simulink subsystem "ACS_Software"  (R2024a)
settings: Solver=VariableStepAuto  StartTime=0.0  StopTime=10.0  RelTol=1e-3
undefined symbols (not defined in the file): epoch, IAU, juliandate, k_Bdot, Kd, km, Kp, m, NoiseStd, s, signQuat, simulator, WMM2020
libraries: sharedtransform x15, simulink_extras x8, aerolibconvert2 x6, matrix_library x5, aerolibutil x5, aerolibtransform2 x2, sharedutil x1, SepehrMILLib x1, aerolibgravity2 x1
(part 1 of 2)
settings Model: Creator=dani  LastModifiedBy=dani

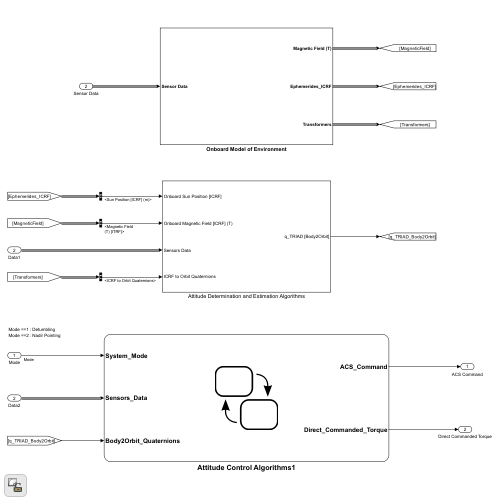
[thumbnail: Simulink's stored preview of the top-level diagram]
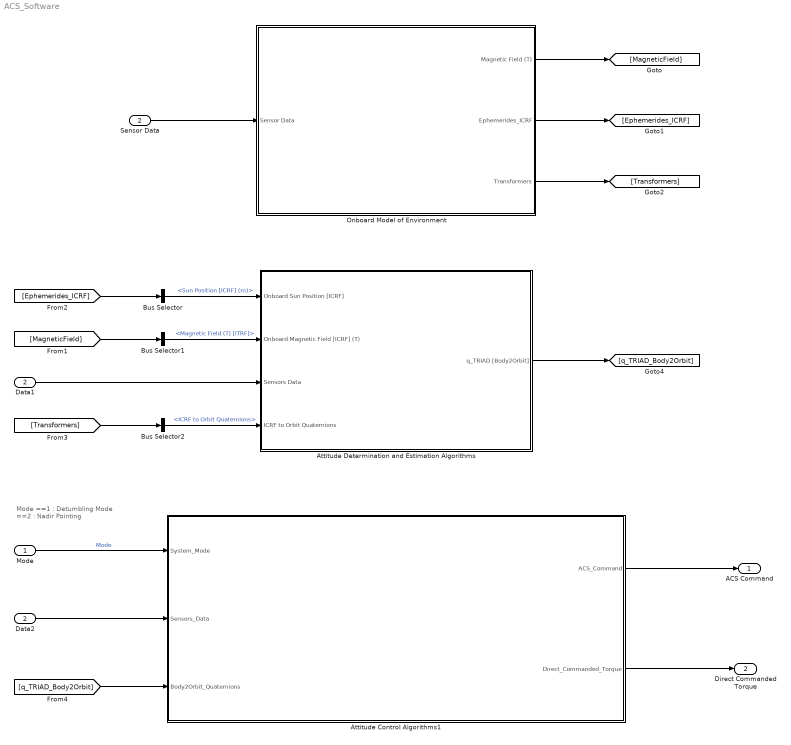
== system ACS_Software ==
  note: Mode ==1 : Detumbling
      | Mode ==2 : Nadir Pointing
  Mode : Inport
  Sensor Data : Inport  Port=2
  Attitude Control Algorithms1 : Stateflow chart  TreatAsAtomicUnit=on
  Attitude Determination and Estimation Algorithms : Subsystem
  Bus Selector : BusSelector  OutputSignals=Sun Ephemeris [ICRF].Sun Position [ICRF] (m)
  Bus Selector1 : BusSelector  OutputSignals=|
      | Magnetic Field
      | (T) [ITRF]
  Bus Selector2 : BusSelector  OutputSignals=Quaternions.ICRF to Orbit Quaternions
  Data1 : InportShadow  Port=2
  Data2 : InportShadow  Port=2
  Onboard Model of Environment : Subsystem
  ACS Command : Outport
  Direct Commanded Torque : Outport  Port=2
  wires:
  Attitude Determination and Estimation Algorithms/1(q_TRIAD [Body2Orbit]) -> [q_TRIAD_Body2Orbit]
  [MagneticField] -> Bus Selector1/1
  Onboard Model of Environment/1(Magnetic Field (T)) -> [MagneticField]
  [Ephemerides_ICRF] -> Bus Selector/1
  Onboard Model of Environment/2(Ephemerides_ICRF) -> [Ephemerides_ICRF]
  Sensor Data/1 -> Onboard Model of Environment/1(Sensor Data)
  Data1/1 -> Attitude Determination and Estimation Algorithms/3(Sensors Data)
  Mode/1 -> Attitude Control Algorithms1/1(System_Mode)  "Mode"
  Attitude Control Algorithms1/1(ACS_Command) -> ACS Command/1
  Data2/1 -> Attitude Control Algorithms1/2(Sensors_Data)
  Bus Selector/1 -> Attitude Determination and Estimation Algorithms/1(Onboard Sun Position [ICRF])  "<Sun Position [ICRF] (m)>"
  Bus Selector1/1 -> Attitude Determination and Estimation Algorithms/2(Onboard Magnetic Field [ICRF] (T))  "<Magnetic Field (T) [ITRF]>"
  Onboard Model of Environment/3(Transformers) -> [Transformers]
  [Transformers] -> Bus Selector2/1
  Bus Selector2/1 -> Attitude Determination and Estimation Algorithms/4(ICRF to Orbit Quaternions)  "<ICRF to Orbit Quaternions>"
  [q_TRIAD_Body2Orbit] -> Attitude Control Algorithms1/3(Body2Orbit_Quaternions)
  Attitude Control Algorithms1/2(Direct_Commanded_Torque) -> Direct Commanded Torque/1

== system ACS_Software/Attitude Control Algorithms1/Detumbling ==
  note: $\frac{k}{||B||}\omega \times B$
  Sensors_Data : Inport
  Action Port : ActionPort
      settings: CopyFcn=Stateflow.SLINSF.SimulinkMan.removeBlockPreDeleteFcn  PreDeleteFcn=Stateflow.SLINSF.SimulinkMan.unsafePredeleteFcn
  Bus Selector1 : BusSelector  OutputSignals=Measured Angular Velocity [Body] (rad/s),Measured Magnetic Field [Body] (T)
  Constant11 : Constant  Value=k_Bdot
  Cross Product : matrix_library/Cross Product
  Divide : Product  Inputs=*/
  Divide1 : Product  Inputs=*/
  Product : Product
  sqrt : Subsystem
  ACS_Command : Outport
  wires:
  sqrt/1(sqrt(u)) -> Divide1/2, Divide/2  "||B||"
  Constant11/1 -> Product/1
  Bus Selector1/2 -> sqrt/1(u), Divide/1  "<Measured Magnetic Field [Body] (T)>"
  Divide/1 -> Cross Product/2  "b"
  Bus Selector1/1 -> Cross Product/1  "<Measured Angular Velocity [Body] (rad/s)>"
  Sensors_Data/1 -> Bus Selector1/1
  Divide1/1 -> ACS_Command/1  "Dipole Command"
  Product/1 -> Divide1/1  "k(omega*b)"
  Cross Product/1 -> Product/2  "omega*b"

== system ACS_Software/Attitude Control Algorithms1/Nadir_Pointing ==
  System_Mode : Inport
  Sensors_Data : Inport  Port=2
  Body2Orbit_Quaternions : Inport  Port=3
  Action Port : ActionPort
      settings: CopyFcn=Stateflow.SLINSF.SimulinkMan.removeBlockPreDeleteFcn  PreDeleteFcn=Stateflow.SLINSF.SimulinkMan.unsafePredeleteFcn
  Nadir Pointing Algorithm : Subsystem
  Terminator : Terminator
  ACS_Command : Outport
  Direct_Commanded_Torque : Outport  Port=2
  wires:
  Sensors_Data/1 -> Nadir Pointing Algorithm/1(Sensors Out)
  Nadir Pointing Algorithm/1(Dipole Command) -> ACS_Command/1  "Dipole Command"
  System_Mode/1 -> Terminator/1
  Nadir Pointing Algorithm/2(Torque Command) -> Direct_Commanded_Torque/1  "Torque Command"
  Body2Orbit_Quaternions/1 -> Nadir Pointing Algorithm/2(Body to Orbit Quaternion)

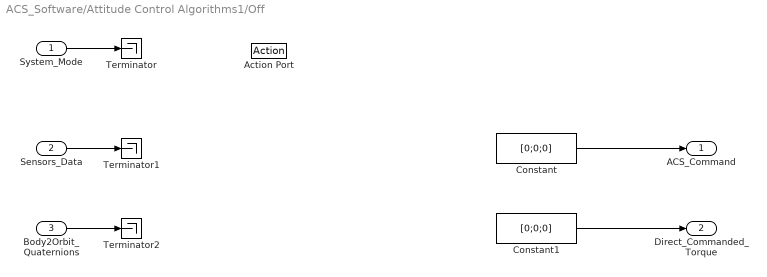
== system ACS_Software/Attitude Control Algorithms1/Off ==
  System_Mode : Inport
  Sensors_Data : Inport  Port=2
  Body2Orbit_Quaternions : Inport  Port=3
  Action Port : ActionPort
      settings: CopyFcn=Stateflow.SLINSF.SimulinkMan.removeBlockPreDeleteFcn  PreDeleteFcn=Stateflow.SLINSF.SimulinkMan.unsafePredeleteFcn
  Constant : Constant  Value=[0;0;0]
  Constant1 : Constant  Value=[0;0;0]
  Terminator : Terminator
  Terminator1 : Terminator
  Terminator2 : Terminator
  ACS_Command : Outport
  Direct_Commanded_Torque : Outport  Port=2
  wires:
  Sensors_Data/1 -> Terminator1/1
  System_Mode/1 -> Terminator/1
  Body2Orbit_Quaternions/1 -> Terminator2/1
  Constant/1 -> ACS_Command/1
  Constant1/1 -> Direct_Commanded_Torque/1

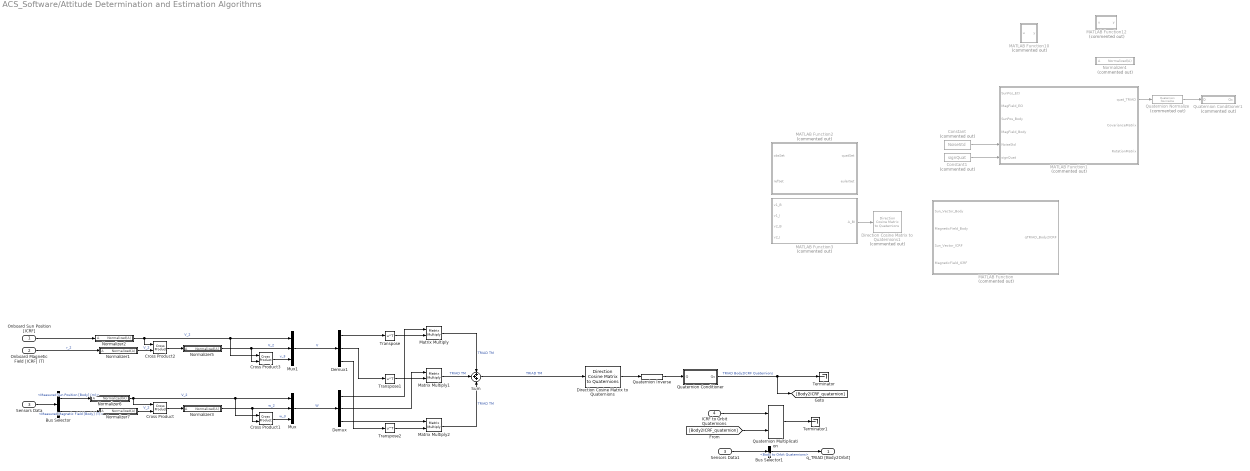
== system ACS_Software/Attitude Determination and Estimation Algorithms ==
  Onboard Sun Position [ICRF] : Inport
  Onboard Magnetic Field [ICRF] (T) : Inport  Port=2
  Sensors Data : Inport  Port=3
  ICRF to Orbit Quaternions : Inport  Port=4
  Bus Selector : BusSelector  OutputSignals=Measured Sun Position [Body] (m),Measured Magnetic Field [Body] (T)
  Bus Selector1 : BusSelector  OutputSignals=Body to Orbit Quaternions
  Constant : Constant  Commented=on  Value=NoiseStd
  Constant1 : Constant  Commented=on  Value=signQuat
  Cross Product{,1..3} (4 alike) : matrix_library/Cross Product
  Demux : Demux  Outputs=3
  Demux1 : Demux  Outputs=3
  Direction Cosine Matrix to Quaternions : sharedtransform/Direction Cosine Matrix  to Quaternions  aMode=0  action=None  tolerance=eps(2)
      settings: LibrarySourceBlock=|
      | aerolibtransform2/Direction Cosine Matrix
      | to Quaternions
  Direction Cosine Matrix to Quaternions1 : sharedtransform/Direction Cosine Matrix  to Quaternions  Commented=on  aMode=0  action=None  tolerance=eps(2)
      settings: LibrarySourceBlock=|
      | aerolibtransform2/Direction Cosine Matrix
      | to Quaternions
  MATLAB Function : MATLAB Function  Commented=on  TreatAsAtomicUnit=on
  MATLAB Function1 : MATLAB Function  Commented=on  TreatAsAtomicUnit=on
  MATLAB Function10 : MATLAB Function  Commented=on  TreatAsAtomicUnit=on
  MATLAB Function12 : MATLAB Function  Commented=on  TreatAsAtomicUnit=on
  MATLAB Function2 : MATLAB Function  Commented=on  TreatAsAtomicUnit=on
  MATLAB Function3 : MATLAB Function  Commented=on  TreatAsAtomicUnit=on
  Matrix Multiply : Product  Multiplication=Matrix(*)
  Matrix Multiply1 : Product  Multiplication=Matrix(*)
  Matrix Multiply2 : Product  Multiplication=Matrix(*)
  Mux : Mux  Inputs=3
  Mux1 : Mux  Inputs=3
  Normalizer1 : Subsystem
  Normalizer2 : Subsystem
  Normalizer3 : Subsystem
  Normalizer4 : Subsystem  Commented=on
  Normalizer5 : Subsystem
  Normalizer6 : Subsystem
  Normalizer7 : Subsystem
  Quaternion Inverse : aerolibutil/Quaternion Inverse
  Quaternion Multiplication : aerolibutil/Quaternion Multiplication
  Quaternion Normalize : sharedutil/Quaternion Normalize  Commented=on  aMode=aMode
  Quaternion Conditioner : Subsystem  TreatAsAtomicUnit=on
      settings: MinAlgLoopOccurrences=on
  Quaternion Conditioner1 : Subsystem  Commented=on  TreatAsAtomicUnit=on
      settings: MinAlgLoopOccurrences=on
  Sensors Data1 : InportShadow  Port=3
  Sum : Sum  Inputs=+++
  Terminator : Terminator
  Terminator1 : Terminator
  Transpose : Math  Operator=transpose
  Transpose1 : Math  Operator=transpose
  Transpose2 : Math  Operator=transpose
  q_TRIAD [Body2Orbit] : Outport
  wires:
  Bus Selector1/1 -> q_TRIAD [Body2Orbit]/1  "<Body to Orbit Quaternions>"
  Sensors Data1/1 -> Bus Selector1/1
  Quaternion Inverse/1 -> Quaternion Conditioner/1(Q)
  Quaternion Multiplication/1 -> Terminator1/1
  [Body2ICRF_quaternion] -> Quaternion Multiplication/2
  ICRF to Orbit Quaternions/1 -> Quaternion Multiplication/1
  Normalizer7/1(Normalized(A)) -> Cross Product/2  "V_2"
  Normalizer6/1(Normalized(A)) -> Mux/1, Cross Product1/1, Cross Product/1  "V_2"
  Normalizer2/1(Normalized(A)) -> Mux1/1, Cross Product3/1, Cross Product2/1  "V_2"
  Normalizer1/1(Normalized(A)) -> Cross Product2/2  "V_2"
  Bus Selector/1 -> Normalizer6/1(A)  "<Measured Sun Position [Body] (m)>"
  Onboard Sun Position [ICRF]/1 -> Normalizer2/1(A)
  Normalizer3/1(Normalized(A)) -> Cross Product1/2, Mux/2  "w_2"
  Onboard Magnetic Field [ICRF] (T)/1 -> Normalizer1/1(A)  "r_2"
  Direction Cosine Matrix to Quaternions/1 -> Quaternion Inverse/1
  Quaternion Conditioner/1(Qc) -> [Body2ICRF_quaternion], Terminator/1  "TRIAD Body2ICRF Quaternions"
  MATLAB Function3/1(A_BI) -> Direction Cosine Matrix to Quaternions1/1
  Matrix Multiply/1 -> Sum/1  "TRIAD TM"
  Matrix Multiply2/1 -> Sum/3  "TRIAD TM"
  Matrix Multiply1/1 -> Sum/2  "TRIAD TM"
  Demux1/1 -> Transpose/1
  Demux1/2 -> Transpose1/1
  Demux/2 -> Matrix Multiply1/1
  Demux1/3 -> Transpose2/1
  Demux/3 -> Matrix Multiply2/1
  Transpose2/1 -> Matrix Multiply2/2
  Transpose1/1 -> Matrix Multiply1/2
  Demux/1 -> Matrix Multiply/1
  Sum/1 -> Direction Cosine Matrix to Quaternions/1  "TRIAD TM"
  Transpose/1 -> Matrix Multiply/2
  Normalizer5/1(Normalized(A)) -> Mux1/2, Cross Product3/2  "V_2"
  Mux1/1 -> Demux1/1  "V"
  Cross Product3/1 -> Mux1/3  "v_3"
  Cross Product2/1 -> Normalizer5/1(A)
  Mux/1 -> Demux/1  "W"
  Cross Product1/1 -> Mux/3  "w_3"
  Cross Product/1 -> Normalizer3/1(A)
  Quaternion Normalize/1 -> Quaternion Conditioner1/1(Q)
  Constant1/1 -> MATLAB Function1/6(signQuat)
  Constant/1 -> MATLAB Function1/5(NoiseStd)
  Bus Selector/2 -> Normalizer7/1(A)  "<Measured Magnetic Field [Body] (T)>"
  Sensors Data/1 -> Bus Selector/1
  MATLAB Function1/1(quat_TRIAD) -> Quaternion Normalize/1

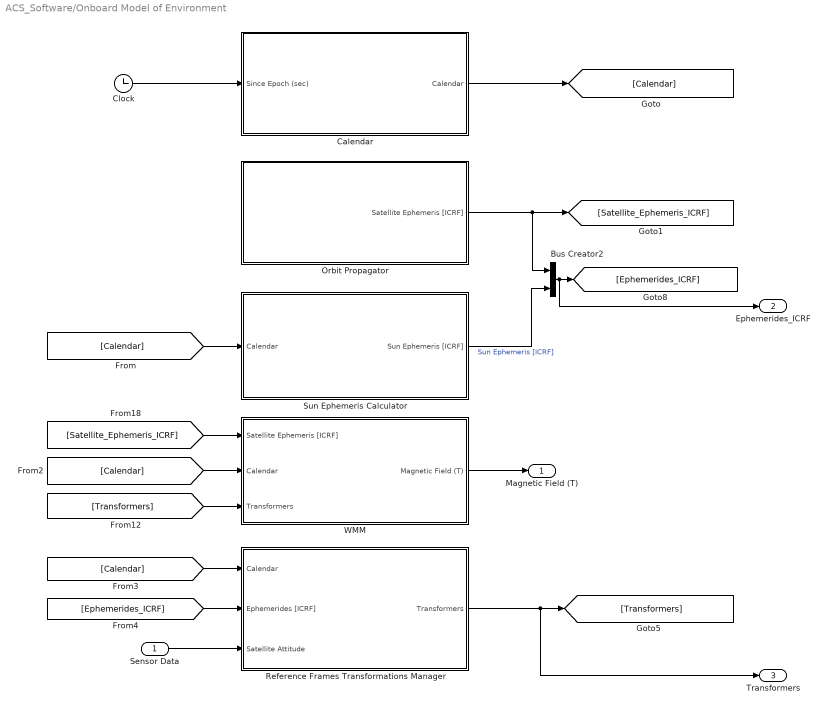
== system ACS_Software/Onboard Model of Environment ==
  Sensor Data : Inport
  Bus Creator2 : BusCreator  Inputs=2
  "Calendar " : Subsystem
  Clock : Clock
  Orbit Propagator : Subsystem
  Reference Frames Transformations Manager : Subsystem
  Sun Ephemeris Calculator : Subsystem
  WMM : Subsystem
  Magnetic Field (T) : Outport
  Ephemerides_ICRF : Outport  Port=2
  Transformers : Outport  Port=3
  wires:
  Sensor Data/1 -> Reference Frames Transformations Manager/3(Satellite Attitude)
  WMM/1(Magnetic Field (T)) -> Magnetic Field (T)/1
  Bus Creator2/1 -> [Ephemerides_ICRF], Ephemerides_ICRF/1
  [Ephemerides_ICRF] -> Reference Frames Transformations Manager/2(Ephemerides [ICRF])
  Clock/1 -> "Calendar "/1(Since Epoch (sec))
  [Calendar] -> Reference Frames Transformations Manager/1(Calendar)
  [Calendar] -> WMM/2(Calendar)
  "Calendar "/1(Calendar) -> [Calendar]
  [Satellite_Ephemeris_ICRF] -> WMM/1(Satellite Ephemeris [ICRF])
  Reference Frames Transformations Manager/1(Transformers) -> [Transformers], Transformers/1
  [Calendar] -> Sun Ephemeris Calculator/1(Calendar)
  Sun Ephemeris Calculator/1(Sun Ephemeris [ICRF]) -> Bus Creator2/2  "Sun Ephemeris [ICRF]"
  Orbit Propagator/1(Satellite Ephemeris [ICRF]) -> [Satellite_Ephemeris_ICRF], Bus Creator2/1
  [Transformers] -> WMM/3(Transformers)

== system ACS_Software/Attitude Control Algorithms1/Detumbling/sqrt ==
  u : Inport
  Dot Product : DotProduct  OutDataTypeStr=Inherit: Inherit via internal rule
  Sqrt1 : Sqrt
  sqrt(u) : Outport
  wires:
  Dot Product/1 -> Sqrt1/1
  u/1 -> Dot Product/2, Dot Product/1
  Sqrt1/1 -> sqrt(u)/1

== system ACS_Software/Attitude Control Algorithms1/Nadir_Pointing/Nadir Pointing Algorithm ==
  Sensors Out : Inport
  Body to Orbit Quaternion : Inport  Port=2
  Bus Selector1 : BusSelector  OutputSignals=Measured Magnetic Field [Body] (T)
  Constant : Constant  Value=[1 ;0 ;0 ;0]
  PD Quaternion Feedback Controller : Subsystem
  q_error Calculator : Subsystem
  Dipole Command : Outport
  Torque Command : Outport  Port=2
  wires:
  Sensors Out/1 -> Bus Selector1/1
  Bus Selector1/1 -> PD Quaternion Feedback Controller/2(B_Body)  "<Measured Magnetic Field [Body] (T)>"
  Constant/1 -> q_error Calculator/1(q_Desired)  "q_Desired"
  PD Quaternion Feedback Controller/1(m_command) -> Dipole Command/1  "m"
  PD Quaternion Feedback Controller/2(T_Command) -> Torque Command/1
  q_error Calculator/1(q_Error) -> PD Quaternion Feedback Controller/1(q_Error)  "q_Error"
  Body to Orbit Quaternion/1 -> q_error Calculator/2(q_Real)

== system ACS_Software/Attitude Determination and Estimation Algorithms/Normalizer1 ==
  A : Inport
  Divide : Product  Inputs=*/
  Dot Product : DotProduct  OutDataTypeStr=Inherit: Inherit via internal rule
  Sqrt1 : Sqrt
  Normalized(A) : Outport
  wires:
  Divide/1 -> Normalized(A)/1
  Sqrt1/1 -> Divide/2
  A/1 -> Dot Product/1, Dot Product/2, Divide/1
  Dot Product/1 -> Sqrt1/1

== system ACS_Software/Attitude Determination and Estimation Algorithms/Normalizer2 ==
  A : Inport
  Divide : Product  Inputs=*/
  Dot Product : DotProduct  OutDataTypeStr=Inherit: Inherit via internal rule
  Sqrt1 : Sqrt
  Normalized(A) : Outport
  wires:
  Sqrt1/1 -> Divide/2
  Divide/1 -> Normalized(A)/1
  A/1 -> Dot Product/1, Dot Product/2, Divide/1
  Dot Product/1 -> Sqrt1/1

== system ACS_Software/Attitude Determination and Estimation Algorithms/Normalizer3 ==
  A : Inport
  Divide : Product  Inputs=*/
  Dot Product : DotProduct  OutDataTypeStr=Inherit: Inherit via internal rule
  Sqrt1 : Sqrt
  Normalized(A) : Outport
  wires:
  Sqrt1/1 -> Divide/2
  Divide/1 -> Normalized(A)/1
  A/1 -> Dot Product/1, Dot Product/2, Divide/1
  Dot Product/1 -> Sqrt1/1

== system ACS_Software/Attitude Determination and Estimation Algorithms/Normalizer4 ==
  A : Inport
  Divide : Product  Inputs=*/
  Dot Product : DotProduct  OutDataTypeStr=Inherit: Inherit via internal rule
  NaNProtection : MATLAB Function  TreatAsAtomicUnit=on
  Sqrt1 : Sqrt
  Normalized(A) : Outport
  wires:
  NaNProtection/1(y) -> Divide/2
  Divide/1 -> Normalized(A)/1
  Sqrt1/1 -> NaNProtection/1(u)
  A/1 -> Dot Product/1, Dot Product/2, Divide/1
  Dot Product/1 -> Sqrt1/1

== system ACS_Software/Attitude Determination and Estimation Algorithms/Normalizer5 ==
  A : Inport
  Divide : Product  Inputs=*/
  Dot Product : DotProduct  OutDataTypeStr=Inherit: Inherit via internal rule
  Sqrt1 : Sqrt
  Normalized(A) : Outport
  wires:
  Divide/1 -> Normalized(A)/1
  Sqrt1/1 -> Divide/2
  A/1 -> Dot Product/1, Dot Product/2, Divide/1
  Dot Product/1 -> Sqrt1/1

== system ACS_Software/Attitude Determination and Estimation Algorithms/Normalizer6 ==
  A : Inport
  Divide : Product  Inputs=*/
  Dot Product : DotProduct  OutDataTypeStr=Inherit: Inherit via internal rule
  Sqrt1 : Sqrt
  Normalized(A) : Outport
  wires:
  Divide/1 -> Normalized(A)/1
  Sqrt1/1 -> Divide/2
  A/1 -> Dot Product/1, Dot Product/2, Divide/1
  Dot Product/1 -> Sqrt1/1

== system ACS_Software/Attitude Determination and Estimation Algorithms/Normalizer7 ==
  A : Inport
  Divide : Product  Inputs=*/
  Dot Product : DotProduct  OutDataTypeStr=Inherit: Inherit via internal rule
  Sqrt1 : Sqrt
  Normalized(A) : Outport
  wires:
  Divide/1 -> Normalized(A)/1
  Sqrt1/1 -> Divide/2
  A/1 -> Dot Product/1, Dot Product/2, Divide/1
  Dot Product/1 -> Sqrt1/1

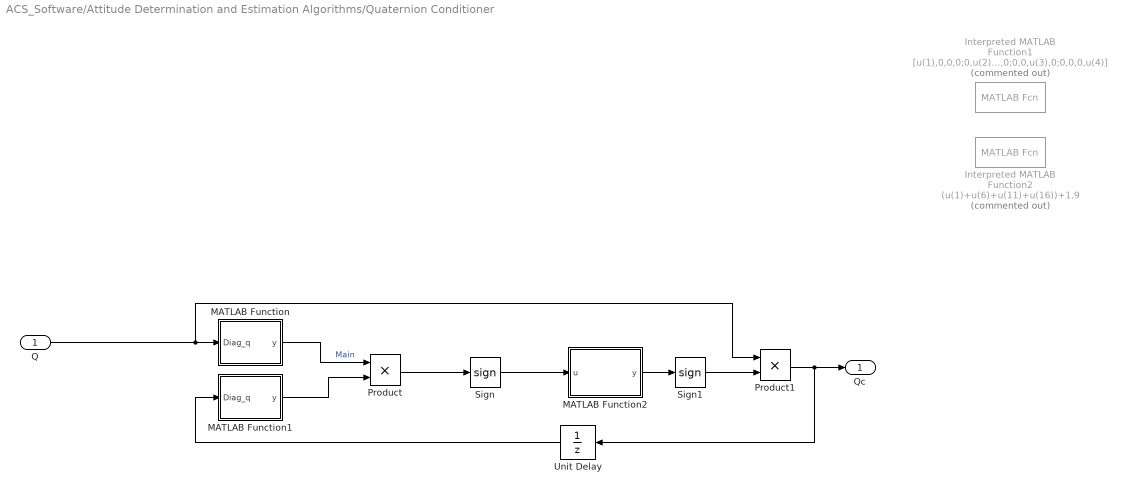
== system ACS_Software/Attitude Determination and Estimation Algorithms/Quaternion Conditioner ==
  Q : Inport  PortDimensions=[4,1]
  Interpreted MATLAB Function1 : MATLABFcn  Commented=on  MATLABFcn=[u(1),0,0,0;0,u(2),0,0;0,0,u(3),0;0,0,0,u(4)]
  Interpreted MATLAB Function2 : MATLABFcn  Commented=on  MATLABFcn=(u(1)+u(6)+u(11)+u(16))+1.9
  MATLAB Function : MATLAB Function  TreatAsAtomicUnit=on
  MATLAB Function1 : MATLAB Function  TreatAsAtomicUnit=on
  MATLAB Function2 : MATLAB Function  TreatAsAtomicUnit=on
  Product : Product
  Product1 : Product
  Sign : Signum
  Sign1 : Signum
  Unit Delay : UnitDelay  InitialCondition=[1;0;0;0]  SampleTime=-1  HasFrameUpgradeWarning=on
  Qc : Outport  PortDimensions=[4,1]
  wires:
  Q/1 -> MATLAB Function/1(Diag_q), Product1/1
  Product1/1 -> Qc/1, Unit Delay/1
  MATLAB Function/1(y) -> Product/1  "Main"
  MATLAB Function2/1(y) -> Sign1/1
  Sign/1 -> MATLAB Function2/1(u)
  Product/1 -> Sign/1
  Sign1/1 -> Product1/2
  MATLAB Function1/1(y) -> Product/2
  Unit Delay/1 -> MATLAB Function1/1(Diag_q)

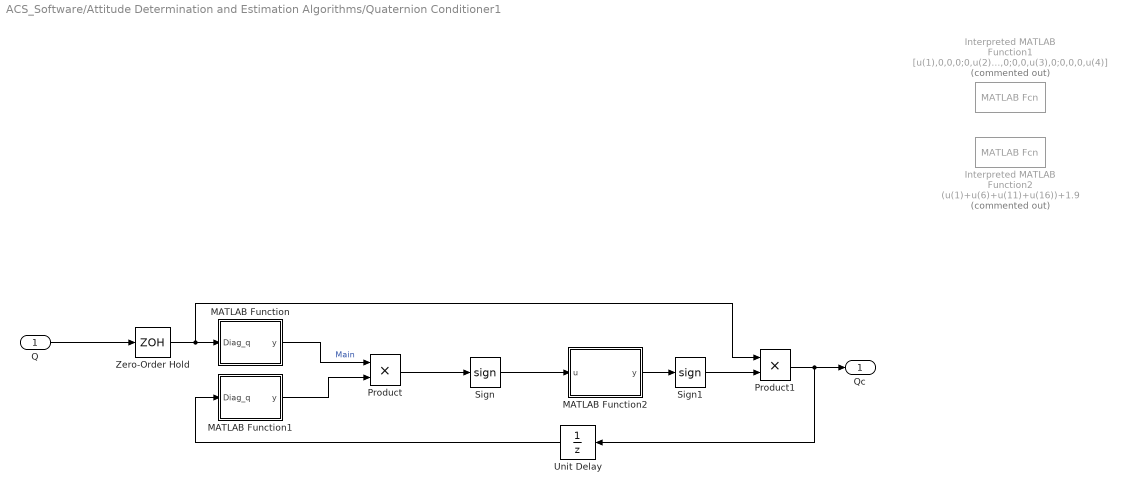
== system ACS_Software/Attitude Determination and Estimation Algorithms/Quaternion Conditioner1 ==
  Q : Inport  PortDimensions=[4,1]
  Interpreted MATLAB Function1 : MATLABFcn  Commented=on  MATLABFcn=[u(1),0,0,0;0,u(2),0,0;0,0,u(3),0;0,0,0,u(4)]
  Interpreted MATLAB Function2 : MATLABFcn  Commented=on  MATLABFcn=(u(1)+u(6)+u(11)+u(16))+1.9
  MATLAB Function : MATLAB Function  TreatAsAtomicUnit=on
  MATLAB Function1 : MATLAB Function  TreatAsAtomicUnit=on
  MATLAB Function2 : MATLAB Function  TreatAsAtomicUnit=on
  Product : Product
  Product1 : Product
  Sign : Signum
  Sign1 : Signum
  Unit Delay : UnitDelay  InitialCondition=[1;0;0;0]  SampleTime=-1  HasFrameUpgradeWarning=on
  Zero-Order Hold : ZeroOrderHold  SampleTime=-1
  Qc : Outport  PortDimensions=[4,1]
  wires:
  Zero-Order Hold/1 -> MATLAB Function/1(Diag_q), Product1/1
  Product1/1 -> Qc/1, Unit Delay/1
  MATLAB Function/1(y) -> Product/1  "Main"
  MATLAB Function2/1(y) -> Sign1/1
  Sign/1 -> MATLAB Function2/1(u)
  Product/1 -> Sign/1
  Sign1/1 -> Product1/2
  Q/1 -> Zero-Order Hold/1
  MATLAB Function1/1(y) -> Product/2
  Unit Delay/1 -> MATLAB Function1/1(Diag_q)

== system ACS_Software/Onboard Model of Environment/Calendar  ==
  Since Epoch (sec) : Inport  OutDataTypeStr=double  Unit=s  PortDimensions=1
  Calendar Bus Creator : BusCreator  Inputs=4
  Constant6 : Constant  Value=epoch.DecimalYear
  JD : Subsystem
  MJD : Subsystem
  Calendar : Outport
  wires:
  MJD/1(Modified Julian Date (day)) -> Calendar Bus Creator/2  "Modified Julian Date (day)"
  Calendar Bus Creator/1 -> Calendar/1  "Calendar_out"
  JD/1(Julian Date (day)) -> Calendar Bus Creator/1  "Julian Date (day)"
  Constant6/1 -> Calendar Bus Creator/3  "Decimal Year (year)"
  Since Epoch (sec)/1 -> Calendar Bus Creator/4, JD/1(Since Epoch (sec)), MJD/1(Since Epoch (sec))  "Since Epoch (sec)"

== system ACS_Software/Onboard Model of Environment/Orbit Propagator ==
  Bus Creator : BusCreator  Inputs=2
  Orbit Propagator Numerical (high precision) : OrbitPropagator  propagator=Numerical (high precision)  startDate=juliandate(epoch.Year, epoch.Month, epoch.Day, epoch.Hour, epoch.Minute, epoch.Second)  dateOut=off  orbitType=Circular inclined  semiMajorAxis=Semi_major_axis  inclination=Inclination  raan=RAAN  argLat=Argument_of_latitude  inertialPosition=[3649700.0 3308200.0 -4676600.0]  inertialVelocity=[-2750.8 6666.4 2573.4]  fixedPosition=[-4142689.0 -2676864.7 -4669861.6]  fixedVelocity=[1452.7 -6720.7 2568.1]  customR=3396200  customMu=4.305e13  customJ2=1.0826269e-03  customOmega=4.06125949e-3
  Satellite Ephemeris [ICRF] : Outport
  wires:
  Orbit Propagator Numerical (high precision)/2 -> Bus Creator/2  "Satellite Velocity [ICRF](m/s)"
  Orbit Propagator Numerical (high precision)/1 -> Bus Creator/1  "Satellite Position [ICRF](m)"
  Bus Creator/1 -> Satellite Ephemeris [ICRF]/1  "Satellite Ephemeris [ICRF]"

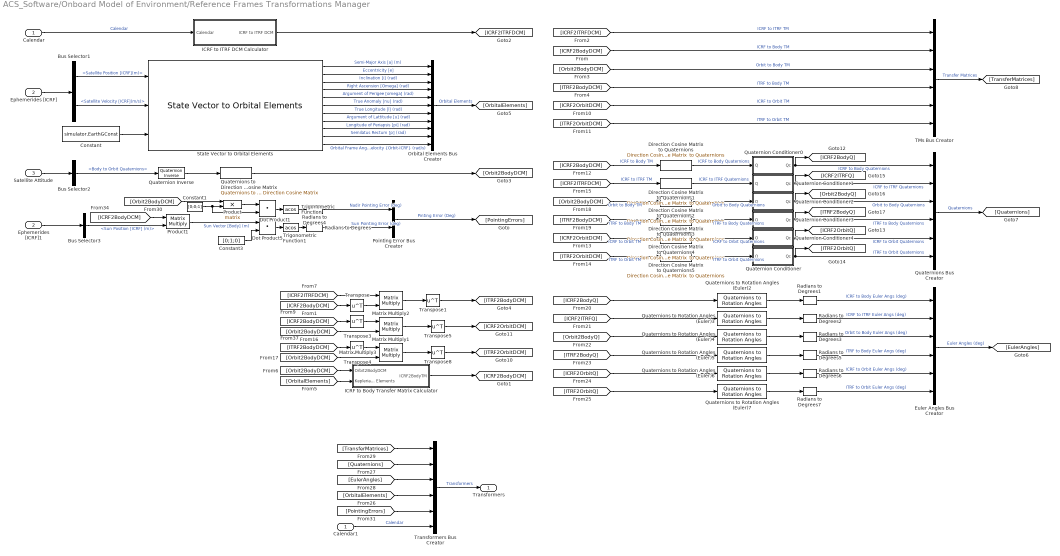
== system ACS_Software/Onboard Model of Environment/Reference Frames Transformations Manager ==
  Calendar : Inport
  Ephemerides [ICRF] : Inport  Port=2
  Satellite Attitude : Inport  Port=3
  Bus Selector1 : BusSelector  OutputSignals=Satellite Ephemeris [ICRF].Satellite Position [ICRF](m),Satellite Ephemeris [ICRF].Satellite Velocity [ICRF](m/s)
  Bus Selector2 : BusSelector  OutputSignals=Body to Orbit Quaternions
  Bus Selector3 : BusSelector  OutputSignals=Sun Ephemeris [ICRF].Sun Position [ICRF] (m)
  Calendar1 : InportShadow
  Constant : Constant  Value=simulator.EarthGConst
  Constant1 : Constant  Value=[0;0;1]
  Constant3 : Constant  Value=[0;1;0]
  Direction Cosine Matrix to Quaternions{,1..5} (6 alike) : sharedtransform/Direction Cosine Matrix  to Quaternions  aMode=0  action=None  tolerance=eps(2)
  Dot Product1 : DotProduct  OutDataTypeStr=Inherit: Inherit via internal rule
  Dot Product5 : DotProduct  OutDataTypeStr=Inherit: Inherit via internal rule
  Ephemerides [ICRF]1 : InportShadow  Port=2
  Euler Angles Bus Creator : BusCreator  Inputs=6
  ICRF to Body Transfer Matrix Calculator : Subsystem
  ICRF to ITRF DCM Calculator : Subsystem
  Matrix Multiply1 : Product  Multiplication=Matrix(*)
  Matrix Multiply2 : Product  Multiplication=Matrix(*)
  Matrix Multiply3 : Product  Multiplication=Matrix(*)
  Orbital Elements Bus Creator : BusCreator  Inputs=11
  Pointing Error Bus Creator : BusCreator  Inputs=2
  Product : Product  Multiplication=Matrix(*)
  Product1 : Product  Multiplication=Matrix(*)
  Quaternion Inverse : aerolibutil/Quaternion Inverse
  Quaternion Conditioner : Subsystem
  Quaternion Conditioner0 : Subsystem
  Quaternion Conditioner1 : Subsystem
  Quaternion Conditioner2 : Subsystem
  Quaternion Conditioner3 : Subsystem
  Quaternion Conditioner4 : Subsystem
  Quaternions Bus Creator : BusCreator  Inputs=6
  Quaternions to Direction Cosine Matrix : sharedtransform/Quaternions to  Direction Cosine Matrix  aMode=aMode
  Quaternions to Rotation Angles (Euler){2..7} (6 alike) : sharedtransform/Quaternions to Rotation Angles  rotationOrder=XYZ  aMode=aMode
  Radians to Degrees{,1..7} (8 alike) : simulink_extras/Transformations/Radians to Degrees
  State Vector to Orbital Elements : SepehrMILLib/Reference Frames Transformations Manager/State Vector to Orbital Elements  SystemSampleTime=-1  VariantActivationTime=update diagram  AllowFlexibleInterface=on  Latency=0  AutoFrameSizeCalculation=off
  TMs Bus Creator : BusCreator  Inputs=6
  Transformers Bus Creator : BusCreator  Inputs=6
  Transpose{,1,3..5,8} (6 alike) : Math  Operator=transpose
  Trigonometric Function : Trigonometry  Operator=acos
  Trigonometric Function1 : Trigonometry  Operator=acos  OutputSignalType=real
  Transformers : Outport
  wires:
  Quaternion Inverse/1 -> Quaternions to Direction Cosine Matrix/1
  Transpose4/1 -> Matrix Multiply3/1
  Transpose8/1 -> [ITRF2OrbitDCM]
  Transpose5/1 -> [ICRF2OrbitDCM]
  [ICRF2BodyDCM] -> Transpose3/1
  Transpose3/1 -> Matrix Multiply1/1
  [Orbit2BodyDCM] -> Matrix Multiply1/2
  Matrix Multiply3/1 -> Transpose8/1
  Matrix Multiply1/1 -> Transpose5/1
  [ITRF2BodyDCM] -> Transpose4/1
  [Orbit2BodyDCM] -> Matrix Multiply3/2
  Radians to Degrees7/1 -> Euler Angles Bus Creator/6  "ITRF to Orbit Euler Angs (deg)"
  Radians to Degrees6/1 -> Euler Angles Bus Creator/5  "ICRF to Orbit Euler Angs (deg)"
  Radians to Degrees5/1 -> Euler Angles Bus Creator/4  "ITRF to Body Euler Angs (deg)"
  Radians to Degrees3/1 -> Euler Angles Bus Creator/3  "Orbit to Body Euler Angs (deg)"
  Radians to Degrees2/1 -> Euler Angles Bus Creator/2  "ICRF to ITRF Euler Angs (deg)"
  Radians to Degrees1/1 -> Euler Angles Bus Creator/1  "ICRF to Body Euler Angs (deg)"
  ICRF to ITRF DCM Calculator/1(ICRF to ITRF DCM) -> [ICRF2ITRFDCM]
  Bus Selector3/1 -> Product1/2  "<Sun Position [ICRF] (m)>"
  [ICRF2BodyDCM] -> Product1/1
  [Orbit2BodyDCM] -> ICRF to Body Transfer Matrix Calculator/1(Orbit2BodyDCM)
  [ICRF2BodyDCM] -> Direction Cosine Matrix to Quaternions/1  "ICRF to Body TM"
  Quaternions to Rotation Angles (Euler)4/1 -> Radians to Degrees3/1
  Trigonometric Function1/1 -> Radians to Degrees/1
  [Orbit2BodyDCM] -> TMs Bus Creator/3  "Orbit to Body TM"
  [ITRF2BodyQ] -> Quaternions to Rotation Angles (Euler)5/1
  Quaternions to Rotation Angles (Euler)6/1 -> Radians to Degrees6/1
  [ICRF2OrbitDCM] -> Direction Cosine Matrix to Quaternions4/1  "ICRF to Orbit TM"
  [TransferMatrices] -> Transformers Bus Creator/1
  State Vector to Orbital Elements/3 -> Orbital Elements Bus Creator/3  "Inclination [i] (rad)"
  Euler Angles Bus Creator/1 -> [EulerAngles]  "Euler Angles (deg)"
  Quaternions to Rotation Angles (Euler)3/1 -> Radians to Degrees2/1
  Quaternions to Rotation Angles (Euler)2/1 -> Radians to Degrees1/1
  Direction Cosine Matrix to Quaternions1/1 -> Quaternion Conditioner1/1(Q)  "ICRF to ITRF Quaternions"
  Dot Product1/1 -> Trigonometric Function/1
  Quaternions to Rotation Angles (Euler)5/1 -> Radians to Degrees5/1
  Quaternion Conditioner0/1(Qc) -> Quaternions Bus Creator/1, [ICRF2BodyQ]  "ICRF to Body Quaternions"
  Direction Cosine Matrix to Quaternions2/1 -> Quaternion Conditioner2/1(Q)  "Orbit to Body Quaternions"
  Quaternion Conditioner3/1(Qc) -> [ITRF2BodyQ], Quaternions Bus Creator/4  "ITRF to Body Quaternions"
  Bus Selector2/1 -> Quaternion Inverse/1  "<Body to Orbit Quaternions>"
  Product/1 -> Dot Product1/1
  Product1/1 -> Dot Product5/1  "Sun Vector [Body] (m)"
  [ITRF2BodyDCM] -> Direction Cosine Matrix to Quaternions3/1  "ITRF to Body TM"
  TMs Bus Creator/1 -> [TransferMatrices]  "Transfer Matrices"
  Direction Cosine Matrix to Quaternions4/1 -> Quaternion Conditioner4/1(Q)  "ICRF to Orbit Quaternions"
  Direction Cosine Matrix to Quaternions5/1 -> Quaternion Conditioner/1(Q)  "ITRF to Orbit Quaternions"
  [ICRF2ITRFDCM] -> Direction Cosine Matrix to Quaternions1/1  "ICRF to ITRF TM"
  Quaternions Bus Creator/1 -> [Quaternions]  "Quaternions"
  Ephemerides [ICRF]/1 -> Bus Selector1/1
  Quaternion Conditioner1/1(Qc) -> [ICRF2ITRFQ], Quaternions Bus Creator/2  "ICRF to ITRF Quaternions"
  State Vector to Orbital Elements/2 -> Orbital Elements Bus Creator/2  "Eccentricity [e]"
  Calendar1/1 -> Transformers Bus Creator/6  "Calendar"
  Satellite Attitude/1 -> Bus Selector2/1
  [ICRF2ITRFDCM] -> Matrix Multiply2/1
  [ITRF2OrbitDCM] -> TMs Bus Creator/6  "ITRF to Orbit TM"
  [Quaternions] -> Transformers Bus Creator/2
  Quaternions to Rotation Angles (Euler)7/1 -> Radians to Degrees7/1
  [ITRF2BodyDCM] -> TMs Bus Creator/4  "ITRF to Body TM"
  Constant1/1 -> Dot Product1/2, Product/2
  [ICRF2BodyQ] -> Quaternions to Rotation Angles (Euler)2/1
  Direction Cosine Matrix to Quaternions3/1 -> Quaternion Conditioner3/1(Q)  "ITRF to Body Quaternions"
  Quaternion Conditioner/1(Qc) -> [ITRF2OrbitQ], Quaternions Bus Creator/6  "ITRF to Orbit Quaternions"
  [ICRF2OrbitDCM] -> TMs Bus Creator/5  "ICRF to Orbit TM"
  Direction Cosine Matrix to Quaternions/1 -> Quaternion Conditioner0/1(Q)  "ICRF to Body Quaternions"
  [Orbit2BodyDCM] -> Product/1
  Transpose/1 -> Matrix Multiply2/2
  [PointingErrors] -> Transformers Bus Creator/5
  [ICRF2BodyDCM] -> TMs Bus Creator/2  "ICRF to Body TM"
  [ICRF2ITRFDCM] -> TMs Bus Creator/1  "ICRF to ITRF TM"
  [Orbit2BodyDCM] -> Direction Cosine Matrix to Quaternions2/1  "Orbit to Body TM"
  Constant/1 -> State Vector to Orbital Elements/3
  State Vector to Orbital Elements/11 -> Orbital Elements Bus Creator/11  "Orbital Frame Angular Velocity {Orbit-ICRF} (rad/s)"
  Pointing Error Bus Creator/1 -> [PointingErrors]  "Pinting Error (Deg)"
  Calendar/1 -> ICRF to ITRF DCM Calculator/1(Calendar)  "Calendar"
  Radians to Degrees/1 -> Pointing Error Bus Creator/2  "Sun Pointing Error (deg)"
  Radians to Degrees4/1 -> Pointing Error Bus Creator/1  "Nadir Pointing Error (deg)"
  [OrbitalElements] -> Transformers Bus Creator/4
  Constant3/1 -> Dot Product5/2
  Trigonometric Function/1 -> Radians to Degrees4/1
  Transpose1/1 -> [ITRF2BodyDCM]
  Orbital Elements Bus Creator/1 -> [OrbitalElements]  "Orbital Elements"
  ICRF to Body Transfer Matrix Calculator/1(ICRF2BodyTM) -> [ICRF2BodyDCM]
  Bus Selector1/1 -> State Vector to Orbital Elements/1  "<Satellite Position [ICRF](m)>"
  Matrix Multiply2/1 -> Transpose1/1
  [ICRF2BodyDCM] -> Transpose/1
  Dot Product5/1 -> Trigonometric Function1/1
  Ephemerides [ICRF]1/1 -> Bus Selector3/1
  [OrbitalElements] -> ICRF to Body Transfer Matrix Calculator/2(Keplerian Elements)
  State Vector to Orbital Elements/1 -> Orbital Elements Bus Creator/1  "Semi-Major Axis [a] (m)"
  Quaternions to Direction Cosine Matrix/1 -> [Orbit2BodyDCM]
  State Vector to Orbital Elements/8 -> Orbital Elements Bus Creator/8  "Argument of Lattitude [u] (rad)"
  Quaternion Conditioner4/1(Qc) -> [ICRF2OrbitQ], Quaternions Bus Creator/5  "ICRF to Orbit Quaternions"
  State Vector to Orbital Elements/9 -> Orbital Elements Bus Creator/9  "Longitude of Periapsis [pi] (rad)"
  State Vector to Orbital Elements/10 -> Orbital Elements Bus Creator/10  "Semilatus Rectum [p] (rad)"
  State Vector to Orbital Elements/4 -> Orbital Elements Bus Creator/4  "Right Ascension [Omega] (rad)"
  Transformers Bus Creator/1 -> Transformers/1  "Transformers"
  State Vector to Orbital Elements/5 -> Orbital Elements Bus Creator/5  "Argument of Perigee [omega] (rad)"
  State Vector to Orbital Elements/6 -> Orbital Elements Bus Creator/6  "True Anomaly [nu] (rad)"
  [EulerAngles] -> Transformers Bus Creator/3
  [ICRF2OrbitQ] -> Quaternions to Rotation Angles (Euler)6/1
  [ICRF2ITRFQ] -> Quaternions to Rotation Angles (Euler)3/1
  Bus Selector1/2 -> State Vector to Orbital Elements/2  "<Satellite Velocity [ICRF](m/s)>"
  [ITRF2OrbitDCM] -> Direction Cosine Matrix to Quaternions5/1  "ITRF to Orbit TM"
  [ITRF2OrbitQ] -> Quaternions to Rotation Angles (Euler)7/1
  [Orbit2BodyQ] -> Quaternions to Rotation Angles (Euler)4/1
  Quaternion Conditioner2/1(Qc) -> [Orbit2BodyQ], Quaternions Bus Creator/3  "Orbit to Body Quaternions"
  State Vector to Orbital Elements/7 -> Orbital Elements Bus Creator/7  "True Longitude [l] (rad)"

== system ACS_Software/Onboard Model of Environment/Sun Ephemeris Calculator ==
  Calendar : Inport
  Bus Selector : BusSelector  OutputSignals=Julian Date (day)
  Length Conversion1 : aerolibconvert2/Length Conversion  IU=km  OU=m
  Sun Ephemeris Bus Creator : BusCreator  Inputs=2
  Sun Ephemeris Calculator : PlanetaryEphem  target=Sun
  Velocity Conversion1 : aerolibconvert2/Velocity Conversion  IU=km/s  OU=m/s
  Sun Ephemeris [ICRF] : Outport
  wires:
  Length Conversion1/1 -> Sun Ephemeris Bus Creator/1  "Sun Position [ICRF] (m)"
  Sun Ephemeris Bus Creator/1 -> Sun Ephemeris [ICRF]/1  "Sun Ephemeris [ICRF]"
  Velocity Conversion1/1 -> Sun Ephemeris Bus Creator/2  "Sun Velocity [ICRF] (m/s)"
  Sun Ephemeris Calculator/2 -> Velocity Conversion1/1
  Sun Ephemeris Calculator/1 -> Length Conversion1/1
  Calendar/1 -> Bus Selector/1
  Bus Selector/1 -> Sun Ephemeris Calculator/1  "<Julian Date (day)>"

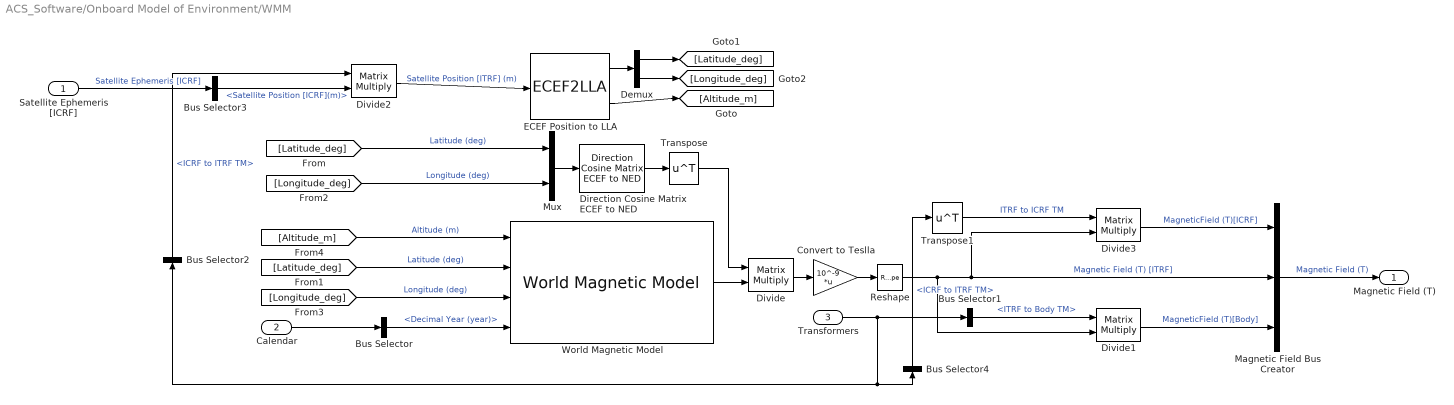
== system ACS_Software/Onboard Model of Environment/WMM ==
  Satellite Ephemeris [ICRF] : Inport
  Calendar : Inport  Port=2
  Transformers : Inport  Port=3
  Bus Selector : BusSelector  OutputSignals=Decimal Year (year)
  Bus Selector1 : BusSelector  OutputSignals=Transfer Matrices.ITRF to Body TM
  Bus Selector2 : BusSelector  OutputSignals=Transfer Matrices.ICRF to ITRF TM
  Bus Selector3 : BusSelector  OutputSignals=Satellite Position [ICRF](m)
  Bus Selector4 : BusSelector  OutputSignals=Transfer Matrices.ICRF to ITRF TM
  Convert to Teslla : Gain  Gain=10^-9  Multiplication=Matrix(K*u)
  Demux : Demux  Outputs=2
  Direction Cosine Matrix ECEF to NED : aerolibtransform2/Direction Cosine Matrix ECEF to NED
  Divide{,1..3} (4 alike) : Product  Inputs=**  Multiplication=Matrix(*)
  ECEF Position to LLA : ECEF2LLA
  Magnetic Field Bus Creator : BusCreator  Inputs=3
  Mux : Mux  Inputs=2
  Reshape : Reshape  OutputDimensionality=Customize  OutputDimensions=[3,1]
  Transpose : Math  Operator=transpose
  Transpose1 : Math  Operator=transpose
  World Magnetic Model : aerolibgravity2/World Magnetic Model  model=WMM2020 (2020-2025)  customFile='WMM2020.COF'  units=Metric (MKS)  time_in=on  month=January  day=1  year=2020  action=Error  h_out=off  dec_out=off  inc_out=off  ti_out=off
  Magnetic Field (T) : Outport
  wires:
  Divide3/1 -> Magnetic Field Bus Creator/1  "MagneticField (T)[ICRF]"
  Transpose1/1 -> Divide3/1  "ITRF to ICRF TM"
  Bus Selector4/1 -> Transpose1/1  "<ICRF to ITRF TM>"
  Bus Selector3/1 -> Divide2/2  "<Satellite Position [ICRF](m)>"
  Bus Selector2/1 -> Divide2/1  "<ICRF to ITRF TM>"
  Satellite Ephemeris [ICRF]/1 -> Bus Selector3/1  "Satellite Ephemeris [ICRF]"
  Bus Selector1/1 -> Divide1/1  "<ITRF to Body TM>"
  World Magnetic Model/1 -> Divide/2
  Divide1/1 -> Magnetic Field Bus Creator/3  "MagneticField (T)[Body]"
  Bus Selector/1 -> World Magnetic Model/4  "<Decimal Year (year)>"
  [Longitude_deg] -> World Magnetic Model/3  "Longitude (deg)"
  Divide2/1 -> ECEF Position to LLA/1  "Satellite Position [ITRF] (m)"
  ECEF Position to LLA/1 -> Demux/1
  Calendar/1 -> Bus Selector/1
  Convert to Teslla/1 -> Reshape/1
  Divide/1 -> Convert to Teslla/1
  Demux/2 -> [Longitude_deg]
  ECEF Position to LLA/2 -> [Altitude_m]
  [Longitude_deg] -> Mux/2  "Longitude (deg)"
  [Latitude_deg] -> Mux/1  "Latitude (deg)"
  Transformers/1 -> Bus Selector4/1, Bus Selector2/1, Bus Selector1/1
  Mux/1 -> Direction Cosine Matrix ECEF to NED/1
  Magnetic Field Bus Creator/1 -> Magnetic Field (T)/1  "Magnetic Field (T)"
  Direction Cosine Matrix ECEF to NED/1 -> Transpose/1
  Reshape/1 -> Divide1/2, Magnetic Field Bus Creator/2, Divide3/2  "Magnetic Field (T) [ITRF]"
  [Altitude_m] -> World Magnetic Model/1  "Altitude (m)"
  Demux/1 -> [Latitude_deg]
  Transpose/1 -> Divide/1
  [Latitude_deg] -> World Magnetic Model/2  "Latitude (deg)"

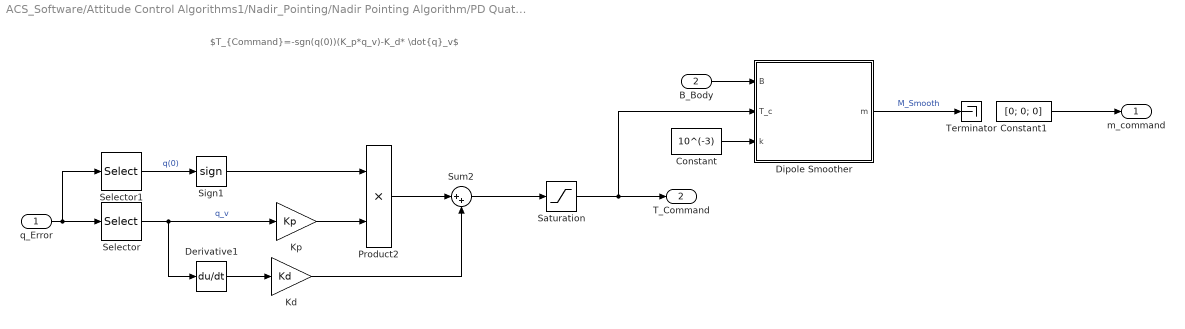
== system ACS_Software/Attitude Control Algorithms1/Nadir_Pointing/Nadir Pointing Algorithm/PD Quaternion Feedback Controller ==
  note: $T_{Command}=-sgn(q(0))(K_p*q_v)-K_d* \dot{q}_v$
  q_Error : Inport
  B_Body : Inport  Port=2
  Constant : Constant  Value=10^(-3)
  Constant1 : Constant  Value=[0; 0; 0]
  Derivative1 : Derivative
  Dipole Smoother : MATLAB Function  TreatAsAtomicUnit=on
  Kd : Gain  Gain=Kd
  Kp : Gain  Gain=Kp
  Product2 : Product
  Saturation : Saturate
  Selector : Selector  InputPortWidth=4  IndexOptions=Index vector (dialog)  Indices=[2 3 4]  OutputSizes=1
  Selector1 : Selector  InputPortWidth=4  IndexOptions=Index vector (dialog)  Indices=[1]  OutputSizes=1
  Sign1 : Signum
  Sum2 : Sum  Inputs=|++
  Terminator : Terminator
  m_command : Outport
  T_Command : Outport  Port=2
  wires:
  q_Error/1 -> Selector1/1, Selector/1
  B_Body/1 -> Dipole Smoother/1(B)
  Selector/1 -> Derivative1/1, Kp/1  "q_v"
  Selector1/1 -> Sign1/1  "q(0)"
  Derivative1/1 -> Kd/1
  Sign1/1 -> Product2/1
  Kd/1 -> Sum2/2
  Product2/1 -> Sum2/1
  Sum2/1 -> Saturation/1
  Kp/1 -> Product2/2
  Constant1/1 -> m_command/1
  Saturation/1 -> T_Command/1, Dipole Smoother/2(T_c)
  Constant/1 -> Dipole Smoother/3(k)
  Dipole Smoother/1(m) -> Terminator/1  "M_Smooth"

== system ACS_Software/Attitude Control Algorithms1/Nadir_Pointing/Nadir Pointing Algorithm/q_error Calculator ==
  note: $q_{Error}=q^{-1}_{Body2Orbit}*q_{Desired}$
  q_Desired : Inport
  q_Real : Inport  Port=2
  Quaternion Inverse : aerolibutil/Quaternion Inverse
  Quaternion Multiplication : aerolibutil/Quaternion Multiplication
  q_Error : Outport
  wires:
  q_Desired/1 -> Quaternion Multiplication/1
  q_Real/1 -> Quaternion Inverse/1
  Quaternion Multiplication/1 -> q_Error/1
  Quaternion Inverse/1 -> Quaternion Multiplication/2

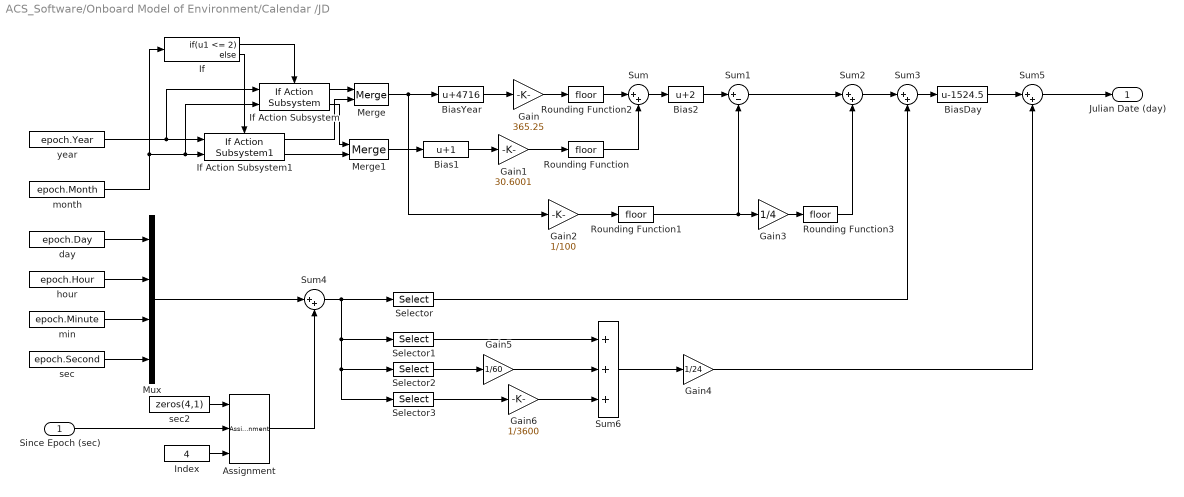
== system ACS_Software/Onboard Model of Environment/Calendar /JD ==
  Since Epoch (sec) : Inport  OutMin=0  PortDimensions=1
  Assignment : Assignment  IndexOptions=Index vector (port)  Indices=1  OutputSizes=1
  Bias1 : Bias  Bias=1  SaturateOnIntegerOverflow=off
  Bias2 : Bias  Bias=2  SaturateOnIntegerOverflow=off
  BiasDay : Bias  Bias=-1524.5  SaturateOnIntegerOverflow=off
  BiasYear : Bias  Bias=4716  SaturateOnIntegerOverflow=off
  Gain : Gain  Gain=365.25
  Gain1 : Gain  Gain=30.6001
  Gain2 : Gain  Gain=1/100
  Gain3 : Gain  Gain=1/4
  Gain4 : Gain  Gain=1/24
  Gain5 : Gain  Gain=1/60
  Gain6 : Gain  Gain=1/3600
  If : If  IfExpression=u1 <= 2
  If Action Subsystem : aerolibconvert2/Julian Date Conversion/If Action Subsystem  SystemSampleTime=-1  VariantActivationTime=update diagram  AllowFlexibleInterface=on  Latency=0  AutoFrameSizeCalculation=off
  If Action Subsystem1 : aerolibconvert2/Julian Date Conversion/If Action Subsystem1  SystemSampleTime=-1  VariantActivationTime=update diagram  AllowFlexibleInterface=on  Latency=0  AutoFrameSizeCalculation=off
  Index : Constant  Value=4
  Merge : Merge
  Merge1 : Merge
  Mux : Mux
  Rounding Function{,1..3} (4 alike) : Rounding
  Selector : Selector  InputPortWidth=4  IndexOptions=Index vector (dialog)  Indices=[1]  OutputSizes=1
  Selector1 : Selector  InputPortWidth=4  IndexOptions=Index vector (dialog)  Indices=[2]  OutputSizes=1
  Selector2 : Selector  InputPortWidth=4  IndexOptions=Index vector (dialog)  Indices=[3]  OutputSizes=1
  Selector3 : Selector  InputPortWidth=4  IndexOptions=Index vector (dialog)  Indices=[4]  OutputSizes=1
  Sum{,2..5} (5 alike) : Sum  Inputs=|++
  Sum1 : Sum  Inputs=|+-
  Sum6 : Sum  Inputs=+++
  day : Constant  Value=epoch.Day
  hour : Constant  Value=epoch.Hour
  min : Constant  Value=epoch.Minute
  month : Constant  Value=epoch.Month
  sec : Constant  Value=epoch.Second
  sec2 : Constant  Value=zeros(4,1)
  year : Constant  Value=epoch.Year
  Julian Date (day) : Outport  VectorParamsAs1DForOutWhenUnconnected=off
  wires:
  Index/1 -> Assignment/3
  If Action Subsystem1/1 -> Merge/2
  min/1 -> Mux/3
  If/1 -> If Action Subsystem/Action
  Selector3/1 -> Gain6/1
  Rounding Function2/1 -> Sum/1
  Selector2/1 -> Gain5/1
  Gain3/1 -> Rounding Function3/1
  Merge/1 -> Gain2/1, BiasYear/1
  BiasYear/1 -> Gain/1
  Gain4/1 -> Sum5/2
  Sum2/1 -> Sum3/1
  Selector1/1 -> Sum6/1
  Sum5/1 -> Julian Date (day)/1
  Sum1/1 -> Sum2/1
  sec2/1 -> Assignment/1
  Gain1/1 -> Rounding Function/1
  Rounding Function3/1 -> Sum2/2
  Bias1/1 -> Gain1/1
  If Action Subsystem/2 -> Merge1/1
  Sum3/1 -> BiasDay/1
  Gain6/1 -> Sum6/3
  year/1 -> If Action Subsystem/1, If Action Subsystem1/1
  If Action Subsystem/1 -> Merge/1
  Sum4/1 -> Selector1/1, Selector2/1, Selector3/1, Selector/1
  Gain2/1 -> Rounding Function1/1
  Gain/1 -> Rounding Function2/1
  Bias2/1 -> Sum1/1
  Assignment/1 -> Sum4/2
  Gain5/1 -> Sum6/2
  Rounding Function1/1 -> Gain3/1, Sum1/2
  If/2 -> If Action Subsystem1/Action
  Since Epoch (sec)/1 -> Assignment/2
  sec/1 -> Mux/4
  Selector/1 -> Sum3/2
  hour/1 -> Mux/2
  BiasDay/1 -> Sum5/1
  Sum6/1 -> Gain4/1
  Sum/1 -> Bias2/1
  If Action Subsystem1/2 -> Merge1/2
  day/1 -> Mux/1
  Rounding Function/1 -> Sum/2
  month/1 -> If Action Subsystem/2, If Action Subsystem1/2, If/1
  Mux/1 -> Sum4/1
  Merge1/1 -> Bias1/1

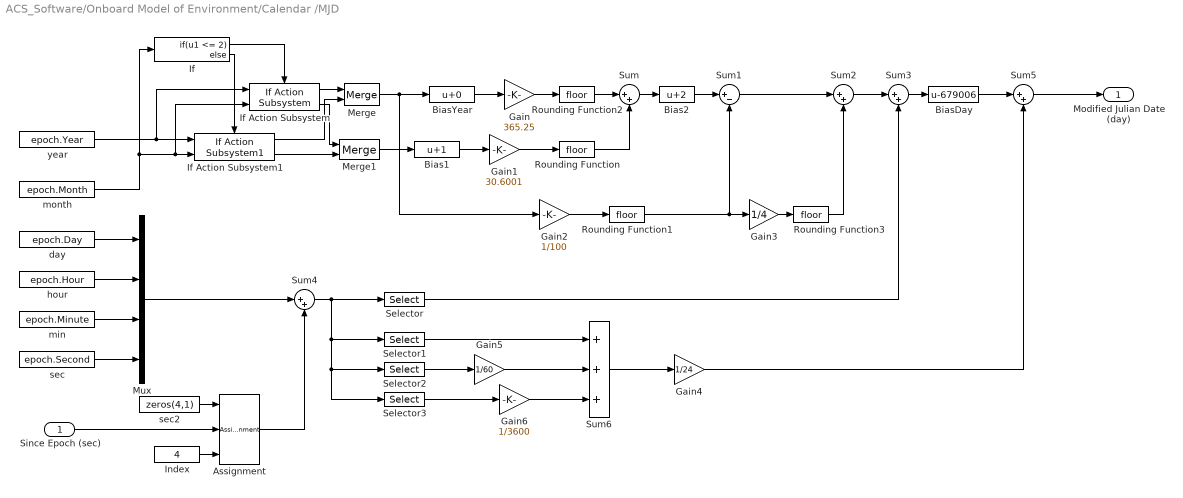
== system ACS_Software/Onboard Model of Environment/Calendar /MJD ==
  Since Epoch (sec) : Inport  OutMin=0  PortDimensions=1
  Assignment : Assignment  IndexOptions=Index vector (port)  Indices=1  OutputSizes=1
  Bias1 : Bias  Bias=1  SaturateOnIntegerOverflow=off
  Bias2 : Bias  Bias=2  SaturateOnIntegerOverflow=off
  BiasDay : Bias  Bias=-679006  SaturateOnIntegerOverflow=off
  BiasYear : Bias  SaturateOnIntegerOverflow=off
  Gain : Gain  Gain=365.25
  Gain1 : Gain  Gain=30.6001
  Gain2 : Gain  Gain=1/100
  Gain3 : Gain  Gain=1/4
  Gain4 : Gain  Gain=1/24
  Gain5 : Gain  Gain=1/60
  Gain6 : Gain  Gain=1/3600
  If : If  IfExpression=u1 <= 2
  If Action Subsystem : aerolibconvert2/Julian Date Conversion/If Action Subsystem  SystemSampleTime=-1  VariantActivationTime=update diagram  AllowFlexibleInterface=on  Latency=0  AutoFrameSizeCalculation=off
  If Action Subsystem1 : aerolibconvert2/Julian Date Conversion/If Action Subsystem1  SystemSampleTime=-1  VariantActivationTime=update diagram  AllowFlexibleInterface=on  Latency=0  AutoFrameSizeCalculation=off
  Index : Constant  Value=4
  Merge : Merge
  Merge1 : Merge
  Mux : Mux
  Rounding Function{,1..3} (4 alike) : Rounding
  Selector : Selector  InputPortWidth=4  IndexOptions=Index vector (dialog)  Indices=[1]  OutputSizes=1
  Selector1 : Selector  InputPortWidth=4  IndexOptions=Index vector (dialog)  Indices=[2]  OutputSizes=1
  Selector2 : Selector  InputPortWidth=4  IndexOptions=Index vector (dialog)  Indices=[3]  OutputSizes=1
  Selector3 : Selector  InputPortWidth=4  IndexOptions=Index vector (dialog)  Indices=[4]  OutputSizes=1
  Sum{,2..5} (5 alike) : Sum  Inputs=|++
  Sum1 : Sum  Inputs=|+-
  Sum6 : Sum  Inputs=+++
  day : Constant  Value=epoch.Day
  hour : Constant  Value=epoch.Hour
  min : Constant  Value=epoch.Minute
  month : Constant  Value=epoch.Month
  sec : Constant  Value=epoch.Second
  sec2 : Constant  Value=zeros(4,1)
  year : Constant  Value=epoch.Year
  Modified Julian Date (day) : Outport  VectorParamsAs1DForOutWhenUnconnected=off
  wires:
  Index/1 -> Assignment/3
  Assignment/1 -> Sum4/2
  If Action Subsystem1/2 -> Merge1/2
  sec/1 -> Mux/4
  month/1 -> If Action Subsystem/2, If Action Subsystem1/2, If/1
  If Action Subsystem/2 -> Merge1/1
  Selector2/1 -> Gain5/1
  If Action Subsystem/1 -> Merge/1
  Merge/1 -> Gain2/1, BiasYear/1
  Sum4/1 -> Selector1/1, Selector2/1, Selector3/1, Selector/1
  If Action Subsystem1/1 -> Merge/2
  Gain5/1 -> Sum6/2
  If/1 -> If Action Subsystem/Action
  Gain3/1 -> Rounding Function3/1
  min/1 -> Mux/3
  Bias1/1 -> Gain1/1
  day/1 -> Mux/1
  sec2/1 -> Assignment/1
  Gain1/1 -> Rounding Function/1
  Rounding Function2/1 -> Sum/1
  Selector3/1 -> Gain6/1
  Sum3/1 -> BiasDay/1
  Rounding Function3/1 -> Sum2/2
  Rounding Function1/1 -> Gain3/1, Sum1/2
  Mux/1 -> Sum4/1
  Gain2/1 -> Rounding Function1/1
  Gain6/1 -> Sum6/3
  Since Epoch (sec)/1 -> Assignment/2
  Merge1/1 -> Bias1/1
  Gain/1 -> Rounding Function2/1
  hour/1 -> Mux/2
  Sum6/1 -> Gain4/1
  Sum5/1 -> Modified Julian Date (day)/1
  year/1 -> If Action Subsystem/1, If Action Subsystem1/1
  Sum1/1 -> Sum2/1
  Selector/1 -> Sum3/2
  BiasDay/1 -> Sum5/1
  Sum2/1 -> Sum3/1
  Sum/1 -> Bias2/1
  Selector1/1 -> Sum6/1
  Bias2/1 -> Sum1/1
  BiasYear/1 -> Gain/1
  Gain4/1 -> Sum5/2
  If/2 -> If Action Subsystem1/Action
  Rounding Function/1 -> Sum/2

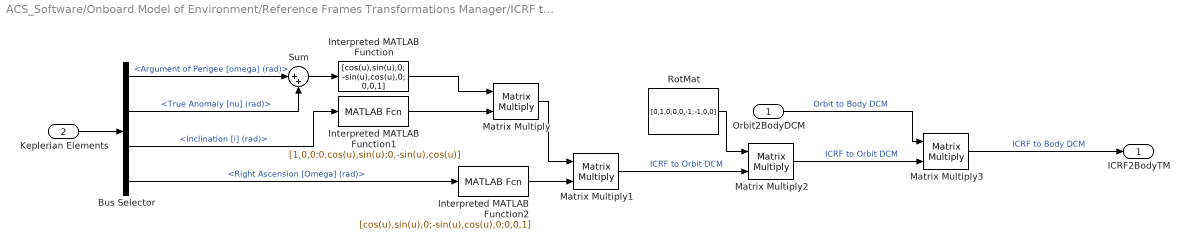
== system ACS_Software/Onboard Model of Environment/Reference Frames Transformations Manager/ICRF to Body Transfer Matrix Calculator ==
  Orbit2BodyDCM : Inport
  Keplerian Elements : Inport  Port=2
  Bus Selector : BusSelector  OutputSignals=Argument of Perigee [omega] (rad),True Anomaly [nu] (rad),Inclination [i] (rad),Right Ascension [Omega] (rad)
  Interpreted MATLAB Function : MATLABFcn  MATLABFcn=[cos(u),sin(u),0; -sin(u),cos(u),0; 0,0,1]  OutputDimensions=[3,3]  Output1D=off
  Interpreted MATLAB Function1 : MATLABFcn  MATLABFcn=[1,0,0;0,cos(u),sin(u);0,-sin(u),cos(u)]  OutputDimensions=[3,3]  Output1D=off
  Interpreted MATLAB Function2 : MATLABFcn  MATLABFcn=[cos(u),sin(u),0;-sin(u),cos(u),0;0,0,1]  OutputDimensions=[3,3]  Output1D=off
  Matrix Multiply{,1..3} (4 alike) : Product  Multiplication=Matrix(*)
  RotMat : Constant  Value=[0,1,0;0,0,-1;-1,0,0]
  Sum : Sum  Inputs=|++
  ICRF2BodyTM : Outport
  wires:
  Matrix Multiply1/1 -> Matrix Multiply2/2  "ICRF to Orbit DCM"
  Bus Selector/4 -> Interpreted MATLAB Function2/1  "<Right Ascension [Omega] (rad)>"
  Interpreted MATLAB Function1/1 -> Matrix Multiply/2
  Matrix Multiply3/1 -> ICRF2BodyTM/1  "ICRF to Body DCM"
  Matrix Multiply/1 -> Matrix Multiply1/1
  Bus Selector/2 -> Sum/2  "<True Anomaly [nu] (rad)>"
  Bus Selector/1 -> Sum/1  "<Argument of Perigee [omega] (rad)>"
  Orbit2BodyDCM/1 -> Matrix Multiply3/1  "Orbit to Body DCM"
  Matrix Multiply2/1 -> Matrix Multiply3/2  "ICRF to Orbit DCM"
  RotMat/1 -> Matrix Multiply2/1
  Sum/1 -> Interpreted MATLAB Function/1
  Interpreted MATLAB Function/1 -> Matrix Multiply/1
  Interpreted MATLAB Function2/1 -> Matrix Multiply1/2
  Keplerian Elements/1 -> Bus Selector/1
  Bus Selector/3 -> Interpreted MATLAB Function1/1  "<Inclination [i] (rad)>"

== system ACS_Software/Onboard Model of Environment/Reference Frames Transformations Manager/ICRF to ITRF DCM Calculator ==
  note: **********************************************************************
      | * *
      | * I E R S B U L L E T I N - A *
      | * *
      | * Rapid Service/Prediction of Earth Orientation *
      | **********************************************************************
      | 30 September 2021 Vol. XXXIV No. 039
      | ______________________________________________________________________
      | GENERAL INFORMATION:
      | To receive this information electronically, contact:
      | ser7@maia.usno.navy.mil or use
      | <http://maia.usno.navy.mil/docrequest.html>
      | MJD = Julian Date - 2 400 000.5 days
      | UT2-UT1 = 0.022 sin(2*pi*T) - 0.012 cos(2*pi*T)
      | - 0.006 sin(4*pi*T) + 0.007 cos(4*pi*T)
      | where pi = 3.14159265... and T is the date in Besselian years.
      | TT = TAI + 32.184 seconds
      | DUT1= (UT1-UTC) transmitted with time signals
      | = -0.1 seconds beginning 17 July 2021 at 0000 UTC
      | Beginning 1 January 2017:
      | TAI-UTC = 37.000 000 seconds
  note: Goal: Transformation Between ICRF (ECI) and ITRF (ECEF)
  Calendar : Inport
  Bus Selector : BusSelector  OutputSignals=Modified Julian Date (day),Since Epoch (sec)
  Constant2 : Constant  Value=37
  Direction Cosine Matrix ICRF to ITRF : aerolibtransform2/Direction Cosine Matrix ECI to ECEF  red=IAU-2000/2006  year=epoch.Year  month=October  day=12  hour=epoch.Hour  min=epoch.Minute  sec=epoch.Second  deltaT=Sec  errorflag=Error  extraparamflag=on
      settings: AttributesFormatString=%<red>
  Earth Orientation Parameters : EOParameters
  ICRF to ITRF DCM : Outport
  wires:
  Bus Selector/2 -> Direction Cosine Matrix ICRF to ITRF/5  "<Since Epoch (sec)>"
  Earth Orientation Parameters/1 -> Direction Cosine Matrix ICRF to ITRF/1
  Bus Selector/1 -> Earth Orientation Parameters/1  "<Modified Julian Date (day)>"
  Direction Cosine Matrix ICRF to ITRF/1 -> ICRF to ITRF DCM/1
  Earth Orientation Parameters/3 -> Direction Cosine Matrix ICRF to ITRF/4  "Celestial Intermediate Pole (CIP)  adjustment (radians)"
  Calendar/1 -> Bus Selector/1
  Constant2/1 -> Direction Cosine Matrix ICRF to ITRF/2
  Earth Orientation Parameters/2 -> Direction Cosine Matrix ICRF to ITRF/3  "Polar Displacement of Earth"

== system ACS_Software/Onboard Model of Environment/Reference Frames Transformations Manager/Quaternion Conditioner ==
  Q : Inport  PortDimensions=[4,1]
  Interpreted MATLAB Function : MATLABFcn  MATLABFcn=[u(1),0,0,0;0,u(2),0,0;0,0,u(3),0;0,0,0,u(4)]
  Interpreted MATLAB Function1 : MATLABFcn  MATLABFcn=[u(1),0,0,0;0,u(2),0,0;0,0,u(3),0;0,0,0,u(4)]
  Interpreted MATLAB Function2 : MATLABFcn  MATLABFcn=(u(1)+u(6)+u(11)+u(16))+1.9
  Product : Product
  Product1 : Product
  Sign : Signum
  Sign1 : Signum
  Unit Delay : UnitDelay  InitialCondition=[1;0;0;0]  SampleTime=-1  HasFrameUpgradeWarning=on
  Qc : Outport  PortDimensions=[4,1]
  wires:
  Unit Delay/1 -> Interpreted MATLAB Function1/1
  Interpreted MATLAB Function1/1 -> Product/2
  Q/1 -> Product1/1, Interpreted MATLAB Function/1
  Sign1/1 -> Product1/2
  Product/1 -> Sign/1
  Sign/1 -> Interpreted MATLAB Function2/1
  Interpreted MATLAB Function2/1 -> Sign1/1
  Interpreted MATLAB Function/1 -> Product/1
  Product1/1 -> Unit Delay/1, Qc/1

== system ACS_Software/Onboard Model of Environment/Reference Frames Transformations Manager/Quaternion Conditioner0 ==
  Q : Inport  PortDimensions=[4,1]
  Interpreted MATLAB Function : MATLABFcn  MATLABFcn=[u(1),0,0,0;0,u(2),0,0;0,0,u(3),0;0,0,0,u(4)]
  Interpreted MATLAB Function1 : MATLABFcn  MATLABFcn=[u(1),0,0,0;0,u(2),0,0;0,0,u(3),0;0,0,0,u(4)]
  Interpreted MATLAB Function2 : MATLABFcn  MATLABFcn=(u(1)+u(6)+u(11)+u(16))+1.9
  Product : Product
  Product1 : Product
  Sign : Signum
  Sign1 : Signum
  Unit Delay : UnitDelay  InitialCondition=[1;0;0;0]  SampleTime=-1  HasFrameUpgradeWarning=on
  Qc : Outport  PortDimensions=[4,1]
  wires:
  Product1/1 -> Qc/1, Unit Delay/1
  Interpreted MATLAB Function/1 -> Product/1
  Interpreted MATLAB Function2/1 -> Sign1/1
  Sign/1 -> Interpreted MATLAB Function2/1
  Product/1 -> Sign/1
  Sign1/1 -> Product1/2
  Q/1 -> Interpreted MATLAB Function/1, Product1/1
  Interpreted MATLAB Function1/1 -> Product/2
  Unit Delay/1 -> Interpreted MATLAB Function1/1

== system ACS_Software/Onboard Model of Environment/Reference Frames Transformations Manager/Quaternion Conditioner1 ==
  Q : Inport  PortDimensions=[4,1]
  Interpreted MATLAB Function : MATLABFcn  MATLABFcn=[u(1),0,0,0;0,u(2),0,0;0,0,u(3),0;0,0,0,u(4)]
  Interpreted MATLAB Function1 : MATLABFcn  MATLABFcn=[u(1),0,0,0;0,u(2),0,0;0,0,u(3),0;0,0,0,u(4)]
  Interpreted MATLAB Function2 : MATLABFcn  MATLABFcn=(u(1)+u(6)+u(11)+u(16))+1.9
  Product : Product
  Product1 : Product
  Sign : Signum
  Sign1 : Signum
  Unit Delay : UnitDelay  InitialCondition=[1;0;0;0]  SampleTime=-1  HasFrameUpgradeWarning=on
  Qc : Outport  PortDimensions=[4,1]
  wires:
  Unit Delay/1 -> Interpreted MATLAB Function1/1
  Interpreted MATLAB Function1/1 -> Product/2
  Q/1 -> Product1/1, Interpreted MATLAB Function/1
  Sign1/1 -> Product1/2
  Product/1 -> Sign/1
  Sign/1 -> Interpreted MATLAB Function2/1
  Interpreted MATLAB Function2/1 -> Sign1/1
  Interpreted MATLAB Function/1 -> Product/1
  Product1/1 -> Unit Delay/1, Qc/1

== system ACS_Software/Onboard Model of Environment/Reference Frames Transformations Manager/Quaternion Conditioner2 ==
  Q : Inport  PortDimensions=[4,1]
  Interpreted MATLAB Function : MATLABFcn  MATLABFcn=[u(1),0,0,0;0,u(2),0,0;0,0,u(3),0;0,0,0,u(4)]
  Interpreted MATLAB Function1 : MATLABFcn  MATLABFcn=[u(1),0,0,0;0,u(2),0,0;0,0,u(3),0;0,0,0,u(4)]
  Interpreted MATLAB Function2 : MATLABFcn  MATLABFcn=(u(1)+u(6)+u(11)+u(16))+1.9
  Product : Product
  Product1 : Product
  Sign : Signum
  Sign1 : Signum
  Unit Delay : UnitDelay  InitialCondition=[1;0;0;0]  SampleTime=-1  HasFrameUpgradeWarning=on
  Qc : Outport  PortDimensions=[4,1]
  wires:
  Product1/1 -> Qc/1, Unit Delay/1
  Interpreted MATLAB Function/1 -> Product/1
  Interpreted MATLAB Function2/1 -> Sign1/1
  Sign/1 -> Interpreted MATLAB Function2/1
  Product/1 -> Sign/1
  Sign1/1 -> Product1/2
  Q/1 -> Interpreted MATLAB Function/1, Product1/1
  Interpreted MATLAB Function1/1 -> Product/2
  Unit Delay/1 -> Interpreted MATLAB Function1/1
